simulink model "sm_car_testrig_bus_VehBusChassisDamper"  (R2022a)
settings: Solver=VariableStepAuto  StartTime=0.0  StopTime=10.0  RelTol=1e-3
libraries: sm_car_lib x3, Dampers_Axle2 x1, fl_lib x1, nesl_utility x1
Description:
  | Copyright 2020-2022 The MathWorks, Inc.
settings Model: Creator=smiller  LastModifiedBy=smiller
settings SolverCC: AlgebraicLoopSolver=TrustRegion
settings DataIOCC: ReturnWorkspaceOutputs=off
settings DebuggingCC: UnconnectedInputMsg=warning  UnconnectedOutputMsg=warning  UnconnectedLineMsg=warning  SFMachineParentedDataDiag=warning  ArithmeticOperatorsInVariantConditions=warning
settings SFSimCC: CustomCodeUndefinedFunction=UseInterfaceOnly
settings RTWCC: DLArmComputeVersion=19.05

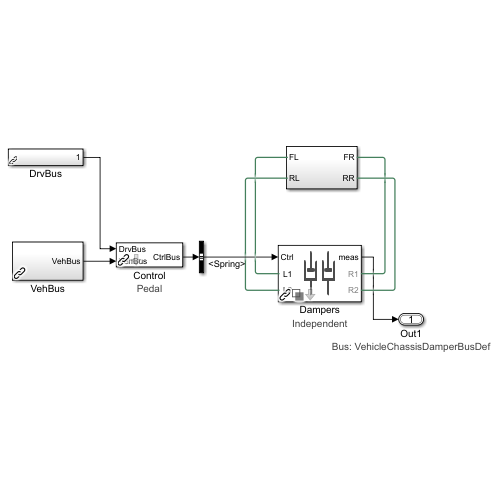
[thumbnail: Simulink's stored preview of the top-level diagram]
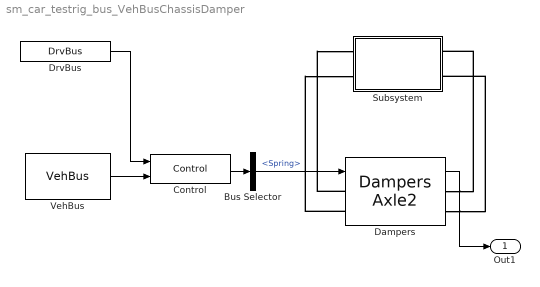
== system sm_car_testrig_bus_VehBusChassisDamper ==
  Bus Selector : BusSelector  OutputSignals=Chassis.Spring
  Control : sm_car_lib/Control/Control  popup_brake_control=Pedal  trq_ratio_front=1
      settings: AttributesFormatString=%<popup_brake_control>
  Dampers : Dampers_Axle2/Dampers Axle2  VariantControl=Variant1  LabelModeActiveChoice=Independent  Damper=Vehicle.Chassis.Damper  VariantLabel=Vehicle.Chassis.Damper.class.Value  InitTriggerDropdown=1
      settings: AttributesFormatString=%<ActiveVariant>
  DrvBus : sm_car_lib/Inputs/DrvBus  SystemSampleTime=-1  VariantActivationTime=update diagram  Latency=0  AutoFrameSizeCalculation=off
  Subsystem : Subsystem
  VehBus : sm_car_lib/Outputs/VehBus  SystemSampleTime=-1  VariantActivationTime=update diagram  Latency=0  AutoFrameSizeCalculation=off
  Out1 : Outport  OutDataTypeStr=Bus: VehicleChassisDamperBusDef  VectorParamsAs1DForOutWhenUnconnected=off
      settings: AttributesFormatString=%<OutDataTypeStr>
  wires:
  Dampers/1 -> Out1/1
  Bus Selector/1 -> Dampers/1  "<Spring>"
  Control/1 -> Bus Selector/1
  DrvBus/1 -> Control/1
  VehBus/1 -> Control/2
  connections:
  Dampers/LConn1 -- Subsystem/LConn1
  Dampers/LConn2 -- Subsystem/LConn2
  Dampers/RConn1 -- Subsystem/RConn1
  Dampers/RConn2 -- Subsystem/RConn2

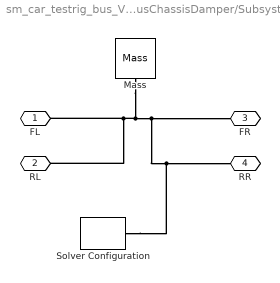
== system sm_car_testrig_bus_VehBusChassisDamper/Subsystem ==
  Mass : fl_lib/Mechanical/Translational Elements/Mass  mass=1 kg  num_ports=foundation.enum.numPorts2.one  v_specify=off  v_priority=High  v=0 m/s  v_nominal_specify=off  v_nominal_unit=m/s  v_nominal_value=1  f_specify=off  f_priority=None  f=0 N  f_nominal_specify=off  f_nominal_unit=N  f_nominal_value=1
      settings: SourceProductBaseCode=PW,SS,VE
  Solver Configuration : nesl_utility/Solver Configuration  PhysicalDomain=network_engine_domain  SubClassName=solver  LeftPortType=input  RightPortType=generic  Tones=[]  Harmonics=[]  SimulateNoise=off  Profile=off  UseLocalSampling=off  EnableSwitchedLinearOptims=on  FrequencyDomain=off  UseCCode=off  RelTol=0.001  AbsTol=1e-06  MinStep=1e-09  ToWorkspace=off  RevertToSquareIcSolve=off  NumHomotopyIterations=100  PhasorMode=off  PhasorModeNumHarmonics=1  IndexReductionMethod=DerivativeReplacement  DoDC=off  ResidualTolerance=1e-09  UseLocalSolver=off  LocalSolverChoice=NE_BACKWARD_EULER_ADVANCER  LocalSolverSampleTime=0.001  DoFixedCost=off  MaxNonlinIter=3  MaxModeIter=2  ComputeImpulses=off  ImpulseIterations=2  LinearAlgebra=auto  LinearAlgebraNumThread=0  EquationFormulation=NE_TIME_EF  DelaysMemoryBudget=1024  AutomaticFiltering=on  FilteringTimeConstant=0.001  PartitionStorageMethod=AS_NEEDED  PartitionMemoryBudget=1024  PartitionMethod=FAST
      settings: SourceProductBaseCode=SS,PW,VE
  FL : PMIOPort  Side=Left
  RL : PMIOPort  Port=2  Side=Left
  FR : PMIOPort  Port=3  Side=Right
  RR : PMIOPort  Port=4  Side=Right
  connections:
  Mass/LConn1 -- Solver Configuration/RConn1 -- RR/RConn1 -- FR/RConn1 -- RL/RConn1 -- FL/RConn1
